simulink model "step_L"  (R2023a)
settings: Solver=VariableStepAuto  StartTime=0.0  StopTime=100  RelTol=1e-3
values from neighbouring files (symbols this model uses):
  ueq = u_eq    [Script_Dirigibile.m]
  x0_tilde = [x0(1)-xeq(1) x0(2)-xeq(2) x0(3)-xeq(3)]    [Script_Dirigibile.m]
  yeq = x_eq    [Script_Dirigibile.m]
undefined symbols (not defined in the file or in its folder): A, B
settings Model: Creator=giuco  LastModifiedBy=giuco

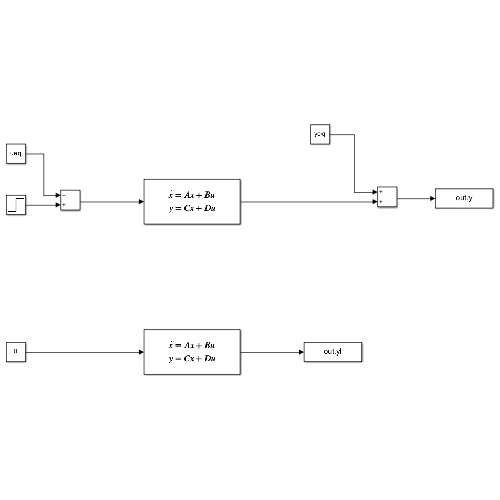
[thumbnail: Simulink's stored preview of the top-level diagram]
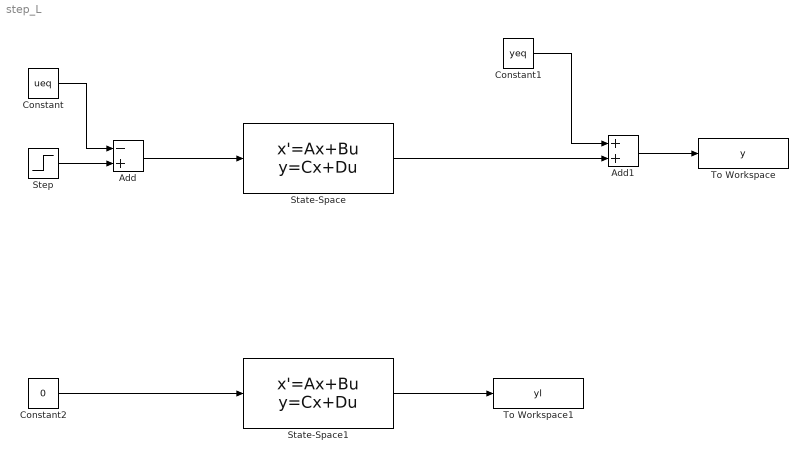
== system step_L ==
  Add : Sum  Inputs=-+
  Add1 : Sum
  Constant : Constant  Value=ueq
  Constant1 : Constant  Value=yeq
  Constant2 : Constant  Value=0
  State-Space : StateSpace  A=A  B=B  C=eye(3)  D=zeros(3,1)  InitialCondition=x0_tilde
  State-Space1 : StateSpace  A=A  B=B  C=eye(3)  D=zeros(3,1)  InitialCondition=x0_tilde
  Step : Step  Time=0  After=1500  SampleTime=0
  To Workspace : ToWorkspace  VariableName=y  SaveFormat=Timeseries  SampleTime=-1
  To Workspace1 : ToWorkspace  VariableName=yl  SaveFormat=Timeseries  SampleTime=-1
  wires:
  Step/1 -> Add/2
  Add/1 -> State-Space/1
  Constant/1 -> Add/1
  Add1/1 -> To Workspace/1
  State-Space/1 -> Add1/2
  Constant1/1 -> Add1/1
  Constant2/1 -> State-Space1/1
  State-Space1/1 -> To Workspace1/1
